simulink model "lfsr"  (R2021a)
settings: Solver=VariableStepAuto  StartTime=0.0  StopTime=10.0  RelTol=1e-3
settings Model: Creator=ANURAG PAL  LastModifiedBy=ANURAG PAL

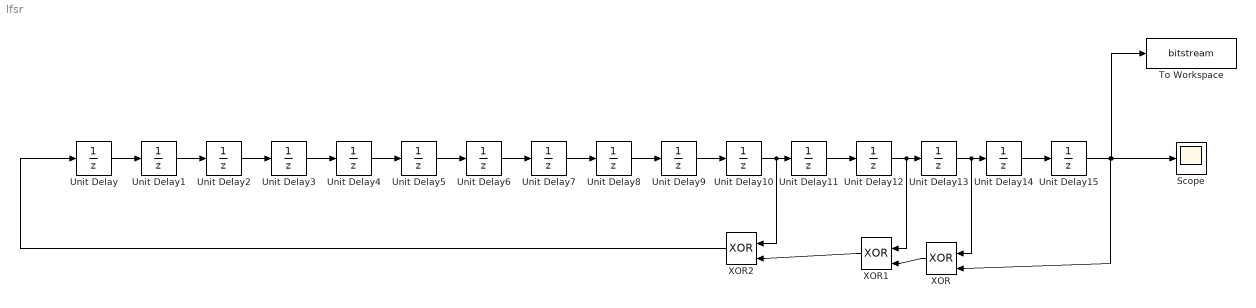
== system lfsr ==
  Scope : Scope
  To Workspace : ToWorkspace  VariableName=bitstream  SampleTime=-1
      settings: MaxDataPoints=10000  Save2DSignal=2-D array (concatenate along first dimension)
  Unit Delay : UnitDelay  InitialCondition=1  SampleTime=-1  HasFrameUpgradeWarning=on
  Unit Delay{1..15} (15 alike) : UnitDelay  SampleTime=-1  HasFrameUpgradeWarning=on
  XOR : Logic  Operator=XOR  IconShape=distinctive  AllPortsSameDT=off  OutDataTypeStr=boolean
  XOR1 : Logic  Operator=XOR  IconShape=distinctive  AllPortsSameDT=off  OutDataTypeStr=boolean
  XOR2 : Logic  Operator=XOR  IconShape=distinctive  AllPortsSameDT=off  OutDataTypeStr=boolean
  wires:
  Unit Delay/1 -> Unit Delay1/1
  Unit Delay3/1 -> Unit Delay4/1
  Unit Delay5/1 -> Unit Delay6/1
  Unit Delay6/1 -> Unit Delay7/1
  Unit Delay9/1 -> Unit Delay10/1
  Unit Delay14/1 -> Unit Delay15/1
  Unit Delay12/1 -> XOR1/1, Unit Delay13/1
  Unit Delay13/1 -> XOR/1, Unit Delay14/1
  Unit Delay11/1 -> Unit Delay12/1
  Unit Delay10/1 -> XOR2/1, Unit Delay11/1
  Unit Delay8/1 -> Unit Delay9/1
  Unit Delay7/1 -> Unit Delay8/1
  Unit Delay4/1 -> Unit Delay5/1
  Unit Delay2/1 -> Unit Delay3/1
  Unit Delay1/1 -> Unit Delay2/1
  XOR/1 -> XOR1/2
  XOR1/1 -> XOR2/2
  XOR2/1 -> Unit Delay/1
  Unit Delay15/1 -> Scope/1, To Workspace/1, XOR/2
